simulink model "sla_fir_filter"  (R2015b)
settings: Solver=FixedStepDiscrete  SolverMode=SingleTasking  StartTime=0.0  StopTime=10.0  RelTol=1e-3
libraries: simulink x2
settings Model: Creator=at-mt  LastModifiedBy=amatsumo
settings DataIOCC: SaveFormat=Array  SignalLoggingSaveFormat=ModelDataLogs  SaveOutput=off  SignalLogging=off  SaveTime=off
settings OptimizationCC: BlockReduction=off  ConditionallyExecuteInputs=off  DefaultParameterBehavior=Inlined  ExpressionDepthLimit=2147483647
settings DebuggingCC: AlgebraicLoopMsg=error  UnderspecifiedInitializationDetection=Classic  MergeDetectMultiDrivingBlocksExec=none  SolverPrmCheckMsg=warning  SingleTaskRateTransMsg=error  FcnCallInpInsideContextMsg=UseLocalSettings  StateNameClashWarn=warning
settings HardwareCC: ProdBitPerPointer=32  ProdLargestAtomicFloat=None  ProdIntDivRoundTo=Undefined  ProdEndianess=Unspecified  ProdWordSize=32  ProdHWDeviceType=ASIC/FPGA->ASIC/FPGA  ProdEqTarget=off
settings GRTTargetCC: GeneratePreprocessorConditionals=Disable all  CombineOutputUpdateFcns=off  GRTInterface=on
settings ConfigComp: CovModelRefEnable=Off  CovSFcnEnable=off

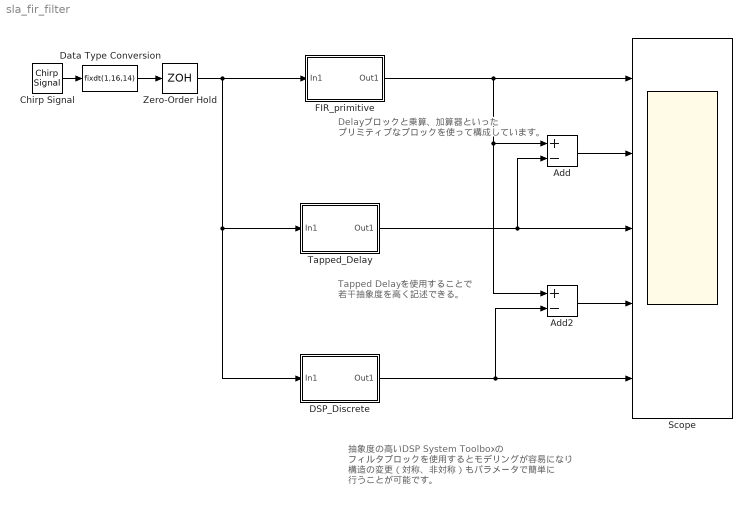
== system sla_fir_filter ==
  note: 抽象度の高いDSP System Toolboxの
      | フィルタブロックを使用するとモデリングが容易になり
      | 構造の変更（対称、非対称）もパラメータで簡単に
      | 行うことが可能です。
  note: Delayブロックと乗算、加算器といった
      | プリミティブなブロックを使って構成しています。
  note: Tapped Delayを使用することで
      | 若干抽象度を高く記述できる。
  Add : Sum  Inputs=+-
  Add2 : Sum  Inputs=+-
  Chirp Signal : simulink/Sources/Chirp Signal  f1=10  T=10  f2=500
  DSP_Discrete : Subsystem
  Data Type Conversion : DataTypeConversion  OutDataTypeStr=fixdt(1,16,14)  RndMeth=Nearest
  FIR_primitive : Subsystem
  Scope : Scope  NumInputPorts=5
  Tapped_Delay : Subsystem
  Zero-Order Hold : ZeroOrderHold  SampleTime=1/1000
  wires:
  Chirp Signal/1 -> Data Type Conversion/1
  Zero-Order Hold/1 -> Tapped_Delay/1(In1), DSP_Discrete/1(In1), FIR_primitive/1(In1)
  FIR_primitive/1(Out1) -> Scope/1, Add/1, Add2/1
  Tapped_Delay/1(Out1) -> Add/2, Scope/3
  Add/1 -> Scope/2
  Data Type Conversion/1 -> Zero-Order Hold/1
  DSP_Discrete/1(Out1) -> Scope/5, Add2/2
  Add2/1 -> Scope/4

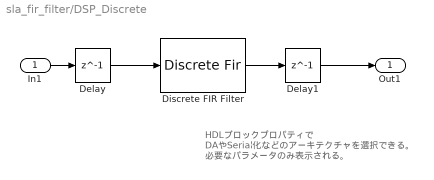
== system sla_fir_filter/DSP_Discrete ==
  note: HDLブロックプロパティで
      | DAやSerial化などのアーキテクチャを選択できる。
      | 必要なパラメータのみ表示される。
  In1 : Inport
  Delay : Delay  DelayLength=1
  Delay1 : Delay  DelayLength=1
  Discrete FIR Filter : DiscreteFir  FilterStructure=Direct form symmetric  Coefficients="[0.02 0.2 0.5 0.2 0.02]  %[0.2 0.3 0.5 0.3 0.2]  %コメント"  InputProcessing=Columns as channels (frame based)  AccumDataTypeStr=fixdt(1,19,14)  RndMeth=Nearest
  Out1 : Outport
  wires:
  Discrete FIR Filter/1 -> Delay1/1
  Delay1/1 -> Out1/1
  In1/1 -> Delay/1
  Delay/1 -> Discrete FIR Filter/1

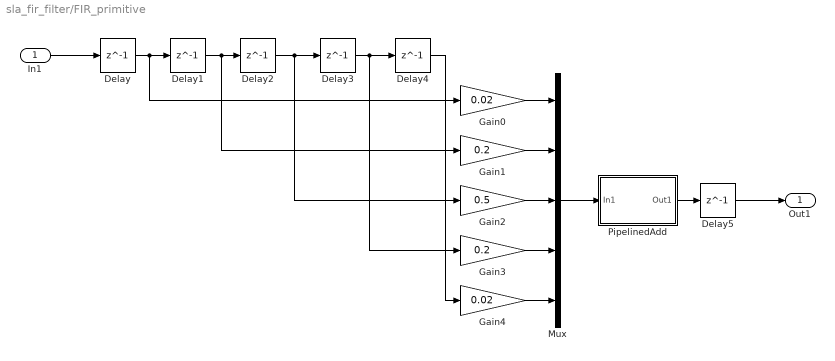
== system sla_fir_filter/FIR_primitive ==
  In1 : Inport
  Delay{,1..5} (6 alike) : Delay  DelayLength=1
  Gain0 : Gain  Gain=0.02  RndMeth=Nearest  OutDataTypeStr=Inherit: Same as input  ParamDataTypeStr=Inherit: Same as input
  Gain1 : Gain  Gain=0.2  RndMeth=Nearest  OutDataTypeStr=Inherit: Same as input  ParamDataTypeStr=Inherit: Same as input
  Gain2 : Gain  Gain=0.5  RndMeth=Nearest  OutDataTypeStr=Inherit: Same as input  ParamDataTypeStr=Inherit: Same as input
  Gain3 : Gain  Gain=0.2  RndMeth=Nearest  OutDataTypeStr=Inherit: Same as input  ParamDataTypeStr=Inherit: Same as input
  Gain4 : Gain  Gain=0.02  RndMeth=Nearest  OutDataTypeStr=Inherit: Same as input  ParamDataTypeStr=Inherit: Same as input
  Mux : Mux  Inputs=5
  PipelinedAdd : Subsystem
  Out1 : Outport
  wires:
  Gain4/1 -> Mux/5
  Gain3/1 -> Mux/4
  Gain2/1 -> Mux/3
  Gain1/1 -> Mux/2
  Gain0/1 -> Mux/1
  Delay4/1 -> Gain4/1
  Delay2/1 -> Delay3/1, Gain2/1
  Delay1/1 -> Delay2/1, Gain1/1
  Delay3/1 -> Delay4/1, Gain3/1
  In1/1 -> Delay/1
  Delay5/1 -> Out1/1
  Delay/1 -> Delay1/1, Gain0/1
  Mux/1 -> PipelinedAdd/1(In1)
  PipelinedAdd/1(Out1) -> Delay5/1

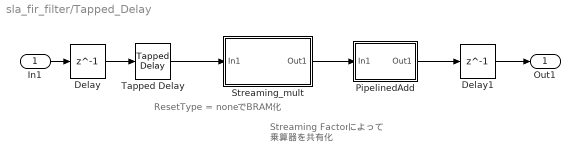
== system sla_fir_filter/Tapped_Delay ==
  note: Streaming Factorによって
      | 乗算器を共有化
  note: ResetType = noneでBRAM化
  In1 : Inport
  Delay : Delay  DelayLength=1
  Delay1 : Delay  DelayLength=1
  PipelinedAdd : Subsystem
  Streaming_mult : Subsystem
  Tapped Delay : simulink/Discrete/Tapped Delay  vinit=0.0  samptime=-1  NumDelays=4  DelayOrder=Oldest  includeCurrent=on
  Out1 : Outport
  wires:
  Tapped Delay/1 -> Streaming_mult/1(In1)
  Streaming_mult/1(Out1) -> PipelinedAdd/1(In1)
  In1/1 -> Delay/1
  PipelinedAdd/1(Out1) -> Delay1/1
  Delay1/1 -> Out1/1
  Delay/1 -> Tapped Delay/1

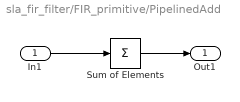
== system sla_fir_filter/FIR_primitive/PipelinedAdd ==
  In1 : Inport
  Sum of Elements : Sum  Inputs=+  RndMeth=Nearest
  Out1 : Outport
  wires:
  Sum of Elements/1 -> Out1/1
  In1/1 -> Sum of Elements/1

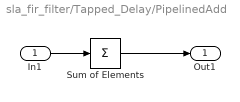
== system sla_fir_filter/Tapped_Delay/PipelinedAdd ==
  In1 : Inport
  Sum of Elements : Sum  Inputs=+  RndMeth=Nearest
  Out1 : Outport
  wires:
  Sum of Elements/1 -> Out1/1
  In1/1 -> Sum of Elements/1

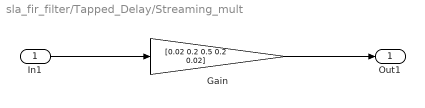
== system sla_fir_filter/Tapped_Delay/Streaming_mult ==
  In1 : Inport
  Gain : Gain  Gain=[0.02 0.2 0.5 0.2 0.02]  RndMeth=Nearest  OutDataTypeStr=Inherit: Same as input  ParamDataTypeStr=Inherit: Same as input
  Out1 : Outport
  wires:
  In1/1 -> Gain/1
  Gain/1 -> Out1/1
